simulink model "adaptivny_tempomat"  (R2023b)
settings: Solver=VariableStepAuto  StartTime=0.0  StopTime=60  RelTol=1e-3
model workspace (MAT data in the model file):
  Maximum_Speed = 25
undefined symbols (not defined in the file): DiscIntNeverNeededParam
libraries: simulink x2, fuzblock x1
settings Model: PacingRate=0.220000  Creator=Vinar  LastModifiedBy=majko
settings OptimizationCC: ReuseModelBlockBuffer=off

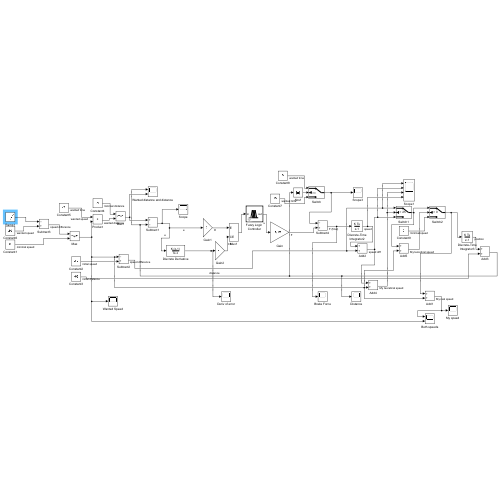
[thumbnail: Simulink's stored preview of the top-level diagram]
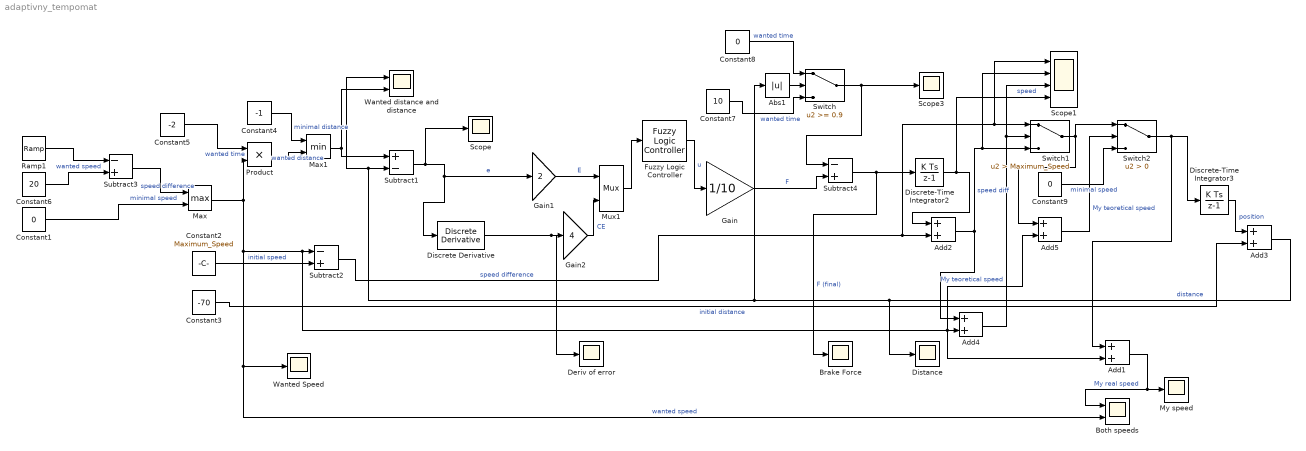
== system adaptivny_tempomat ==
  Abs1 : Abs  SaturateOnIntegerOverflow=off
  Add{1..5} (5 alike) : Sum
  Both speeds : Scope  NumInputPorts=2
  Brake Force : Scope
  Constant1 : Constant  Value=0
  Constant2 : Constant  Value=Maximum_Speed
  Constant3 : Constant  Value=-70
  Constant4 : Constant  Value=-1
  Constant5 : Constant  Value=-2
  Constant6 : Constant  Value=20
  Constant7 : Constant  Value=10
  Constant8 : Constant  Value=0
  Constant9 : Constant  Value=0
  Deriv of error : Scope
  Discrete Derivative : simulink/Discrete/Discrete Derivative  gainval=1.0  ICPrevScaledInput=300  OutMin=[]  OutMax=[]  OutDataType=fixdt(1, 16)  OutScaling=2^-10  DoSatur=off
  Discrete-Time Integrator2 : DiscreteIntegrator  SampleTime=0.1  ICPrevOutput=DiscIntNeverNeededParam  ICPrevScaledInput=DiscIntNeverNeededParam
  Discrete-Time Integrator3 : DiscreteIntegrator  SampleTime=0.1  ICPrevOutput=DiscIntNeverNeededParam  ICPrevScaledInput=DiscIntNeverNeededParam
  Distance : Scope
  Fuzzy Logic Controller : fuzblock/Fuzzy Logic  Controller  FIS='fuzzy_controller.fis'  OutputSampleNumber=101  DataType=double  FuzzifiedInputs=off  RuleFiringStrengths=off  RuleOutputs=off  AggregatedOutputs=off  SimulateUsing=Interpreted execution  OutOfRangeInputValueMessage=warning  NoRuleFiredMessage=warning  EmptyOutputFuzzySetMessage=warning
  Gain : Gain  Gain=1/10
  Gain1 : Gain  Gain=2
  Gain2 : Gain  Gain=4
  Max : MinMax  Function=max  Inputs=2
  Max1 : MinMax  Inputs=2
  Mux1 : Mux  Inputs=2
      settings: DisplayOption=signals
  My speed : Scope
  Product : Product
  Ramp1 : simulink/Sources/Ramp  slope=-0.5  start=0  InitialOutput=0
  Scope : Scope
  Scope1 : Scope  NumInputPorts=4
  Scope3 : Scope
  Subtract1 : Sum  Inputs=+-
  Subtract2 : Sum  Inputs=-+
  Subtract3 : Sum  Inputs=-+
  Subtract4 : Sum  Inputs=-+
  Switch : Switch  Threshold=0.9  SaturateOnIntegerOverflow=off  InputSameDT=off
  Switch1 : Switch  Criteria=u2 > Threshold  Threshold=Maximum_Speed  SaturateOnIntegerOverflow=off  InputSameDT=off
  Switch2 : Switch  Criteria=u2 > Threshold  SaturateOnIntegerOverflow=off  InputSameDT=off
  Wanted Speed : Scope
  Wanted distance and distance : Scope  NumInputPorts=2
  wires:
  Subtract1/1 -> Scope/1, Gain1/1, Discrete Derivative/1  "e"
  Gain1/1 -> Mux1/1  "E"
  Gain2/1 -> Mux1/2  "CE"
  Mux1/1 -> Fuzzy Logic Controller/1
  Gain/1 -> Subtract4/2  "F"
  Discrete-Time Integrator2/1 -> Scope1/4, Add2/1  "speed"
  Discrete-Time Integrator3/1 -> Add3/1  "position"
  Add3/1 -> Distance/1, Subtract1/2, Wanted distance and distance/1, Abs1/1  "distance"
  Constant2/1 -> Subtract2/2  "initial speed"
  Constant3/1 -> Add3/2  "initial distance"
  Fuzzy Logic Controller/1 -> Gain/1  "u"
  Constant5/1 -> Product/1  "wanted time"
  Max/1 -> Product/2, Both speeds/2, Wanted Speed/1, Add1/2, Add4/2, Add5/2, Subtract2/1  "wanted speed"
  Subtract2/1 -> Add2/2, Scope1/1, Switch1/1  "speed difference"
  Add4/1 -> Scope1/3, Switch1/2  "My teoretical speed"
  Constant6/1 -> Subtract3/2  "wanted speed"
  Ramp1/1 -> Subtract3/1
  Subtract3/1 -> Max/1  "speed difference"
  Constant1/1 -> Max/2  "minimal speed"
  Product/1 -> Max1/2  "wanted distance"
  Constant4/1 -> Max1/1  "minimal distance"
  Max1/1 -> Wanted distance and distance/2, Subtract1/1
  Switch/1 -> Subtract4/1, Scope3/1
  Subtract4/1 -> Brake Force/1, Discrete-Time Integrator2/1  "F (final)"
  Discrete Derivative/1 -> Deriv of error/1, Gain2/1
  Add2/1 -> Scope1/2, Switch1/3, Add4/1  "speed diff"
  Add1/1 -> Both speeds/1, My speed/1  "My real speed"
  Abs1/1 -> Switch/2
  Constant8/1 -> Switch/1  "wanted time"
  Constant7/1 -> Switch/3  "wanted time"
  Switch1/1 -> Switch2/1, Add5/1
  Switch2/1 -> Add1/1, Discrete-Time Integrator3/1
  Constant9/1 -> Switch2/3  "minimal speed"
  Add5/1 -> Switch2/2  "My teoretical speed"
